simulink model "optimized_airport_sim_2"  (R2021a)
settings: Solver=VariableStepAuto  StartTime=0.0  StopTime=1e5  RelTol=1e-3
undefined symbols (not defined in the file): m, n
(part 2 of 2)

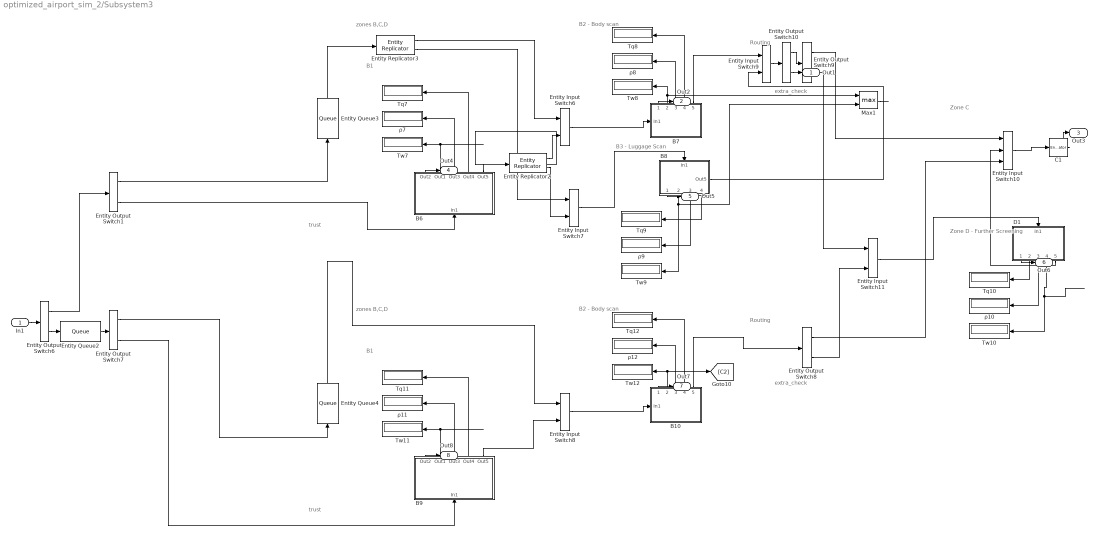
== system optimized_airport_sim_2/Subsystem3 ==
  note: B1
  note: zones B,C,D
  note: Zone C
  note: B3 -
      | Luggage
      | Scan
  note: Routing
  note: Zone D -
      |
      | Further
      | Screening
  note: B2 -
      | Body
      | scan
  note: trust
  note: extra_check
  note: B1
  note: zones B,C,D
  note: Routing
  note: B2 -
      | Body
      | scan
  note: trust
  note: extra_check
  In1 : Inport
  B10 : Subsystem
      settings: PortSchema="{\"entries\":[{\"content\":{\"sides\":[{\"content\":{\"connectorIds\":[]},\"type\":\"ConnectorPlacement.EquallySpacedRectSide\",\"uuid\":\"7ea955c4-59a0-4b16-a665-3c7419b36f79\"},{\"content\":{\"connectorIds\":[\"Out1\",\"Out2\",\"Out3\",\"Out4\",\"Out5\"],\"side\":\"RIGHT\"},\"type\":\"ConnectorPlacement.EquallySpacedRectSide\",\"uuid\":\"a8a3c229-e196-4360-bdfa-8ef645b2ce9c\"},{\"content\":{\"connectorIds\":[\"In1\"],\"side\":\"TOP\"},\"type\":\"ConnectorPlacement.EquallySpacedRectSide\",\"uuid\":\"5260f7b5-f6e8-463a-b0c5-598c56357d98\"}]},\"type\":\"ConnectorPlacement.EquallySpacedConnector\",\"uuid\":\"58c66fb9-1797-41d8-b8ed-62a065428871\"}],\"packageUris\":[\"http://schema.mathworks.com/mf0/Connector/R2020b\"],\"version\":\"1.0\"}"
  B6 : Subsystem
  B7 : Subsystem
      settings: PortSchema="{\"entries\":[{\"content\":{\"sides\":[{\"content\":{\"connectorIds\":[]},\"type\":\"ConnectorPlacement.EquallySpacedRectSide\",\"uuid\":\"7ea955c4-59a0-4b16-a665-3c7419b36f79\"},{\"content\":{\"connectorIds\":[\"Out1\",\"Out2\",\"Out3\",\"Out4\",\"Out5\"],\"side\":\"RIGHT\"},\"type\":\"ConnectorPlacement.EquallySpacedRectSide\",\"uuid\":\"a8a3c229-e196-4360-bdfa-8ef645b2ce9c\"},{\"content\":{\"connectorIds\":[\"In1\"],\"side\":\"TOP\"},\"type\":\"ConnectorPlacement.EquallySpacedRectSide\",\"uuid\":\"5260f7b5-f6e8-463a-b0c5-598c56357d98\"}]},\"type\":\"ConnectorPlacement.EquallySpacedConnector\",\"uuid\":\"58c66fb9-1797-41d8-b8ed-62a065428871\"}],\"packageUris\":[\"http://schema.mathworks.com/mf0/Connector/R2020b\"],\"version\":\"1.0\"}"
  B8 : Subsystem
      settings: PortSchema="{\"entries\":[{\"content\":{\"sides\":[{\"content\":{\"connectorIds\":[\"In1\"]},\"type\":\"ConnectorPlacement.EquallySpacedRectSide\",\"uuid\":\"7ea955c4-59a0-4b16-a665-3c7419b36f79\"},{\"content\":{\"connectorIds\":[\"Out1\",\"Out2\",\"Out3\",\"Out4\"],\"side\":\"RIGHT\"},\"type\":\"ConnectorPlacement.EquallySpacedRectSide\",\"uuid\":\"a8a3c229-e196-4360-bdfa-8ef645b2ce9c\"},{\"content\":{\"connectorIds\":[],\"side\":\"TOP\"},\"type\":\"ConnectorPlacement.EquallySpacedRectSide\",\"uuid\":\"5260f7b5-f6e8-463a-b0c5-598c56357d98\"},{\"content\":{\"connectorIds\":[\"Out5\"],\"side\":\"BOTTOM\"},\"type\":\"ConnectorPlacement.EquallySpacedRectSide\",\"uuid\":\"b778f381-c9da-4203-8e39-7c353a561693\"}]},\"type\":\"ConnectorPlacement.EquallySpacedConnector\",\"uuid\":\"58c66fb9-1797-41d8-b8ed-62a065428871\"}],\"packageUris\":[\"http://schema.mathworks.com/mf0/Connector/R2020b\"],\"version\":\"1.0\"}"
  B9 : Subsystem
  C1 : EntityTerminator  InputPortMessageModes=m  NumberEntitiesArrived=on
      settings: OutputPortMap=o0
  D1 : Subsystem
  Entity Input Switch10 : EntityInputSwitch  InputPortMessageModes=m,m,m  OutputPortMessageModes=m  NumberInputPorts=3  SwitchingCriterion=Equiprobable  Seed=450279
      settings: InputPortMap=u1,u2,u3
  Entity Input Switch11 : EntityInputSwitch  InputPortMessageModes=m,m  OutputPortMessageModes=m  SwitchingCriterion=Equiprobable  Seed=450279
  Entity Input Switch6 : EntityInputSwitch  InputPortMessageModes=m,m  OutputPortMessageModes=m
  Entity Input Switch7 : EntityInputSwitch  InputPortMessageModes=m,m  OutputPortMessageModes=m
  Entity Input Switch8 : EntityInputSwitch  InputPortMessageModes=m,m  OutputPortMessageModes=m
  Entity Input Switch9 : EntityInputSwitch  InputPortMessageModes=m,m  OutputPortMessageModes=m  ActivePortSelection=Switch  SwitchingCriterion=Equiprobable  Seed=450279
  Entity Output Switch1 : EntityOutputSwitch  InputPortMessageModes=m  OutputPortMessageModes=m,m  SwitchingCriterion=From attribute  Seed=9647085  SwitchAttributeName=trust
  Entity Output Switch10 : EntityOutputSwitch  InputPortMessageModes=m  OutputPortMessageModes=m,m  SwitchingCriterion=Equiprobable  Seed=604377
  Entity Output Switch6 : EntityOutputSwitch  InputPortMessageModes=m  OutputPortMessageModes=m,m  SwitchingCriterion=From attribute  Seed=9647085  SwitchAttributeName=luggage
  Entity Output Switch7 : EntityOutputSwitch  InputPortMessageModes=m  OutputPortMessageModes=m,m  SwitchingCriterion=From attribute  Seed=9647085  SwitchAttributeName=trust
  Entity Output Switch8 : EntityOutputSwitch  InputPortMessageModes=m  OutputPortMessageModes=m,m  SwitchingCriterion=From attribute  Seed=9632160  SwitchAttributeName=extra_check
  Entity Output Switch9 : EntityOutputSwitch  InputPortMessageModes=m  OutputPortMessageModes=m,m  SwitchingCriterion=From attribute  Seed=9632160  SwitchAttributeName=extra_check
  Entity Queue2 : Queue  InputPortMessageModes=m  OutputPortMessageModes=m  Capacity=Inf
  Entity Queue3 : Queue  InputPortMessageModes=m  OutputPortMessageModes=m  Capacity=inf
  Entity Queue4 : Queue  InputPortMessageModes=m  OutputPortMessageModes=m  Capacity=inf
  Entity Replicator2 : EntityReplicator  InputPortMessageModes=m  OutputPortMessageModes=m,m
  Entity Replicator3 : EntityReplicator  InputPortMessageModes=m  OutputPortMessageModes=m,m
  Max1 : MinMax  Function=max  Inputs=2
  Tq{7..12} (6 alike) : Display
  Tw{7..12} (6 alike) : Display
  ρ{7..12} (6 alike) : Display
  Out1 : Outport
  Out2 : Outport  Port=2
  Out3 : Outport  Port=3
  Out4 : Outport  Port=4
  Out5 : Outport  Port=5
  Out6 : Outport  Port=6
  Out7 : Outport  Port=7
  Out8 : Outport  Port=8
  wires:
  B10/4(Out4) -> Tq12/1
  B8/3(Out3) -> ρ9/1
  Entity Output Switch8/1 -> Entity Input Switch10/3
  C1/1 -> Out3/1
  Entity Output Switch1/2 -> B6/1(In1)
  Entity Input Switch10/1 -> C1/1
  B7/2(Out1) -> Tw8/1, Max1/1
  B10/5(Out5) -> Entity Output Switch8/1
  Max1/1 -> ?
  Entity Input Switch9/1 -> Entity Output Switch10/1
  Entity Output Switch9/2 -> Entity Input Switch11/1
  D1/5(Out5) -> Entity Input Switch10/2
  B8/5(Out5) -> Entity Input Switch9/2
  Entity Input Switch11/1 -> D1/1(In1)
  B9/2(Out1) -> Tw11/1
  Entity Output Switch8/2 -> Entity Input Switch11/2
  B10/3(Out3) -> ρ12/1
  B6/5(Out5) -> Entity Replicator2/1
  B10/2(Out1) -> Tw12/1, [C2]
  Entity Input Switch8/1 -> B10/1(In1)
  B9/4(Out4) -> Tq11/1
  Entity Replicator3/2 -> Entity Input Switch7/1
  D1/1(Out2) -> Out6/1
  B6/2(Out1) -> Tw7/1
  B9/3(Out3) -> ρ11/1
  B9/5(Out5) -> Entity Input Switch8/2
  Entity Queue4/1 -> Entity Input Switch8/1
  B6/1(Out2) -> Out4/1
  D1/3(Out3) -> ρ10/1
  Entity Input Switch7/1 -> B8/1(In1)
  Entity Replicator2/2 -> Entity Input Switch7/2
  D1/4(Out4) -> Tw10/1
  Entity Replicator2/1 -> Entity Input Switch6/2
  Entity Queue3/1 -> Entity Replicator3/1
  Entity Input Switch6/1 -> B7/1(In1)
  B8/1(Out2) -> Out5/1
  B8/2(Out1) -> Max1/2, Tw9/1
  Entity Replicator3/1 -> Entity Input Switch6/1
  B7/3(Out3) -> ρ8/1
  D1/2(Out1) -> Tq10/1
  B9/1(Out2) -> Out8/1
  B6/3(Out3) -> ρ7/1
  Entity Output Switch9/1 -> Entity Input Switch10/1
  B10/1(Out2) -> Out7/1
  B8/4(Out4) -> Tq9/1
  B7/5(Out5) -> Entity Input Switch9/1
  B6/4(Out4) -> Tq7/1
  Entity Output Switch10/1 -> Entity Output Switch9/1
  B7/4(Out4) -> Tq8/1
  Entity Output Switch10/2 -> Out1/1
  B7/1(Out2) -> Out2/1
  Entity Output Switch1/1 -> Entity Queue3/1
  Entity Output Switch7/1 -> Entity Queue4/1
  Entity Output Switch6/2 -> Entity Queue2/1
  Entity Output Switch6/1 -> Entity Output Switch1/1
  Entity Output Switch7/2 -> B9/1(In1)
  Entity Queue2/1 -> Entity Output Switch7/1
  In1/1 -> Entity Output Switch6/1

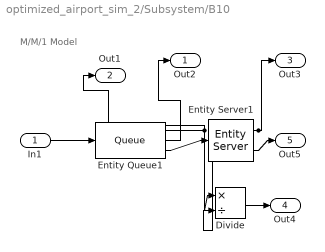
== system optimized_airport_sim_2/Subsystem/B10 ==
  note: M/M/1 Model
  In1 : Inport
  Divide : Product  Inputs=*/
  Entity Queue1 : Queue  InputPortMessageModes=m  OutputPortMessageModes=n,n,m  Capacity=inf  AverageWait=on  AverageQueueLength=on
      settings: OutputPortMap=o2,o3,o5
  Entity Server1 : EntityServer  InputPortMessageModes=m  OutputPortMessageModes=n,m  Capacity=1  ServiceTimeSource=MATLAB action  ServiceTimeAction=|  Utilization=on
      | dt = rand(1,1);
      | persistent rngInit;
      | if isempty(rngInit)
      |     seed = 7612432;
      |     rng(seed);
      |     rngInit = true;
      | end
      | 
      | % Pattern: Exponential distribution
      | mu = 7;
      | dt = -mu * log(1 - rand());
      settings: OutputPortMap=o5,o9
  Out2 : Outport
  Out1 : Outport  Port=2
  Out3 : Outport  Port=3
  Out4 : Outport  Port=4
  Out5 : Outport  Port=5
  wires:
  Divide/1 -> Out4/1
  Entity Server1/2 -> Out5/1
  Entity Queue1/3 -> Entity Server1/1
  Entity Queue1/1 -> Out1/1, Divide/1
  Entity Server1/1 -> Out3/1, Divide/2
  Entity Queue1/2 -> Out2/1
  In1/1 -> Entity Queue1/1

== system optimized_airport_sim_2/Subsystem/B6 ==
  note: M/M/1 Model
  In1 : Inport
  Divide : Product  Inputs=*/
  Entity Queue1 : Queue  InputPortMessageModes=m  OutputPortMessageModes=n,n,m  Capacity=inf  AverageWait=on  AverageQueueLength=on
      settings: OutputPortMap=o2,o3,o5
  Entity Server1 : EntityServer  InputPortMessageModes=m  OutputPortMessageModes=n,m  Capacity=1  ServiceTimeSource=MATLAB action  ServiceTimeAction=|  Utilization=on
      | dt = rand(1,1);
      | persistent rngInit;
      | if isempty(rngInit)
      |     seed = 2273520;
      |     rng(seed);
      |     rngInit = true;
      | end
      | 
      | % Pattern: Exponential distribution
      | mu = 15;
      | dt = -mu * log(1 - rand());
      settings: OutputPortMap=o5,o9
  Out2 : Outport
  Out1 : Outport  Port=2
  Out3 : Outport  Port=3
  Out4 : Outport  Port=4
  Out5 : Outport  Port=5
  wires:
  Divide/1 -> Out4/1
  Entity Server1/2 -> Out5/1
  Entity Queue1/3 -> Entity Server1/1
  Entity Queue1/1 -> Out1/1, Divide/1
  Entity Server1/1 -> Out3/1, Divide/2
  Entity Queue1/2 -> Out2/1
  In1/1 -> Entity Queue1/1

== system optimized_airport_sim_2/Subsystem/B7 ==
  note: M/M/1 Model
  In1 : Inport
  Divide : Product  Inputs=*/
  Entity Queue1 : Queue  InputPortMessageModes=m  OutputPortMessageModes=n,n,m  Capacity=inf  AverageWait=on  AverageQueueLength=on
      settings: OutputPortMap=o2,o3,o5
  Entity Server1 : EntityServer  InputPortMessageModes=m  OutputPortMessageModes=n,m  Capacity=1  ServiceTimeSource=MATLAB action  ServiceTimeAction=|  Utilization=on
      | dt = rand(1,1);
      | persistent rngInit;
      | if isempty(rngInit)
      |     seed = 7612432;
      |     rng(seed);
      |     rngInit = true;
      | end
      | 
      | % Pattern: Exponential distribution
      | mu = 7;
      | dt = -mu * log(1 - rand());
      settings: OutputPortMap=o5,o9
  Out2 : Outport
  Out1 : Outport  Port=2
  Out3 : Outport  Port=3
  Out4 : Outport  Port=4
  Out5 : Outport  Port=5
  wires:
  In1/1 -> Entity Queue1/1
  Entity Queue1/2 -> Out2/1
  Entity Server1/1 -> Divide/2, Out3/1
  Entity Queue1/1 -> Divide/1, Out1/1
  Entity Queue1/3 -> Entity Server1/1
  Entity Server1/2 -> Out5/1
  Divide/1 -> Out4/1

== system optimized_airport_sim_2/Subsystem/B8 ==
  note: M/M/1 Model
  In1 : Inport
  Divide : Product  Inputs=*/
  Entity Queue1 : Queue  InputPortMessageModes=m  OutputPortMessageModes=n,n,m  Capacity=inf  AverageWait=on  AverageQueueLength=on
      settings: OutputPortMap=o2,o3,o5
  Entity Server1 : EntityServer  InputPortMessageModes=m  OutputPortMessageModes=n,m  Capacity=1  ServiceTimeSource=MATLAB action  ServiceTimeAction=|  Utilization=on
      | dt = rand(1,1);
      | persistent rngInit;
      | if isempty(rngInit)
      |     seed = 6069205;
      |     rng(seed);
      |     rngInit = true;
      | end
      | 
      | % Pattern: Exponential distribution
      | mu = 8;
      | dt = -mu * log(1 - rand());
      settings: OutputPortMap=o5,o9
  Out2 : Outport
  Out1 : Outport  Port=2
  Out3 : Outport  Port=3
  Out4 : Outport  Port=4
  Out5 : Outport  Port=5
  wires:
  Divide/1 -> Out4/1
  Entity Server1/2 -> Out5/1
  Entity Queue1/3 -> Entity Server1/1
  Entity Queue1/1 -> Out1/1, Divide/1
  Entity Server1/1 -> Out3/1, Divide/2
  Entity Queue1/2 -> Out2/1
  In1/1 -> Entity Queue1/1

== system optimized_airport_sim_2/Subsystem/B9 ==
  note: M/M/1 Model
  In1 : Inport
  Divide : Product  Inputs=*/
  Entity Queue1 : Queue  InputPortMessageModes=m  OutputPortMessageModes=n,n,m  Capacity=inf  AverageWait=on  AverageQueueLength=on
      settings: OutputPortMap=o2,o3,o5
  Entity Server1 : EntityServer  InputPortMessageModes=m  OutputPortMessageModes=n,m  Capacity=1  ServiceTimeSource=MATLAB action  ServiceTimeAction=|  Utilization=on
      | dt = rand(1,1);
      | persistent rngInit;
      | if isempty(rngInit)
      |     seed = 2273520;
      |     rng(seed);
      |     rngInit = true;
      | end
      | 
      | % Pattern: Exponential distribution
      | mu = 10;
      | dt = -mu * log(1 - rand());
      settings: OutputPortMap=o5,o9
  Out2 : Outport
  Out1 : Outport  Port=2
  Out3 : Outport  Port=3
  Out4 : Outport  Port=4
  Out5 : Outport  Port=5
  wires:
  In1/1 -> Entity Queue1/1
  Entity Queue1/2 -> Out2/1
  Entity Server1/1 -> Divide/2, Out3/1
  Entity Queue1/1 -> Divide/1, Out1/1
  Entity Queue1/3 -> Entity Server1/1
  Entity Server1/2 -> Out5/1
  Divide/1 -> Out4/1

== system optimized_airport_sim_2/Subsystem/D1 ==
  note: M/M/1 Model
  In1 : Inport
  Divide : Product  Inputs=*/
  Entity Queue1 : Queue  InputPortMessageModes=m  OutputPortMessageModes=n,n,m  Capacity=inf  AverageWait=on  AverageQueueLength=on
      settings: OutputPortMap=o2,o3,o5
  Entity Server1 : EntityServer  InputPortMessageModes=m  OutputPortMessageModes=n,m  Capacity=1  ServiceTimeSource=MATLAB action  ServiceTimeAction=|  Utilization=on
      | dt = rand(1,1);
      | persistent rngInit;
      | if isempty(rngInit)
      |     seed = 6069205;
      |     rng(seed);
      |     rngInit = true;
      | end
      | 
      | % Pattern: Exponential distribution
      | mu = 60*3;
      | dt = -mu * log(1 - rand());
      settings: OutputPortMap=o5,o9
  Out2 : Outport
  Out1 : Outport  Port=2
  Out3 : Outport  Port=3
  Out4 : Outport  Port=4
  Out5 : Outport  Port=5
  wires:
  In1/1 -> Entity Queue1/1
  Entity Queue1/2 -> Out2/1
  Entity Server1/1 -> Divide/2, Out3/1
  Entity Queue1/1 -> Divide/1, Out1/1
  Entity Queue1/3 -> Entity Server1/1
  Entity Server1/2 -> Out5/1
  Divide/1 -> Out4/1

== system optimized_airport_sim_2/Subsystem1/B10 ==
  note: M/M/1 Model
  In1 : Inport
  Divide : Product  Inputs=*/
  Entity Queue1 : Queue  InputPortMessageModes=m  OutputPortMessageModes=n,n,m  Capacity=inf  AverageWait=on  AverageQueueLength=on
      settings: OutputPortMap=o2,o3,o5
  Entity Server1 : EntityServer  InputPortMessageModes=m  OutputPortMessageModes=n,m  Capacity=1  ServiceTimeSource=MATLAB action  ServiceTimeAction=|  Utilization=on
      | dt = rand(1,1);
      | persistent rngInit;
      | if isempty(rngInit)
      |     seed = 7612432;
      |     rng(seed);
      |     rngInit = true;
      | end
      | 
      | % Pattern: Exponential distribution
      | mu = 7;
      | dt = -mu * log(1 - rand());
      settings: OutputPortMap=o5,o9
  Out2 : Outport
  Out1 : Outport  Port=2
  Out3 : Outport  Port=3
  Out4 : Outport  Port=4
  Out5 : Outport  Port=5
  wires:
  In1/1 -> Entity Queue1/1
  Entity Queue1/2 -> Out2/1
  Entity Server1/1 -> Divide/2, Out3/1
  Entity Queue1/1 -> Divide/1, Out1/1
  Entity Queue1/3 -> Entity Server1/1
  Entity Server1/2 -> Out5/1
  Divide/1 -> Out4/1

== system optimized_airport_sim_2/Subsystem1/B6 ==
  note: M/M/1 Model
  In1 : Inport
  Divide : Product  Inputs=*/
  Entity Queue1 : Queue  InputPortMessageModes=m  OutputPortMessageModes=n,n,m  Capacity=inf  AverageWait=on  AverageQueueLength=on
      settings: OutputPortMap=o2,o3,o5
  Entity Server1 : EntityServer  InputPortMessageModes=m  OutputPortMessageModes=n,m  Capacity=1  ServiceTimeSource=MATLAB action  ServiceTimeAction=|  Utilization=on
      | dt = rand(1,1);
      | persistent rngInit;
      | if isempty(rngInit)
      |     seed = 2273520;
      |     rng(seed);
      |     rngInit = true;
      | end
      | 
      | % Pattern: Exponential distribution
      | mu = 15;
      | dt = -mu * log(1 - rand());
      settings: OutputPortMap=o5,o9
  Out2 : Outport
  Out1 : Outport  Port=2
  Out3 : Outport  Port=3
  Out4 : Outport  Port=4
  Out5 : Outport  Port=5
  wires:
  In1/1 -> Entity Queue1/1
  Entity Queue1/2 -> Out2/1
  Entity Server1/1 -> Divide/2, Out3/1
  Entity Queue1/1 -> Divide/1, Out1/1
  Entity Queue1/3 -> Entity Server1/1
  Entity Server1/2 -> Out5/1
  Divide/1 -> Out4/1

== system optimized_airport_sim_2/Subsystem1/B7 ==
  note: M/M/1 Model
  In1 : Inport
  Divide : Product  Inputs=*/
  Entity Queue1 : Queue  InputPortMessageModes=m  OutputPortMessageModes=n,n,m  Capacity=inf  AverageWait=on  AverageQueueLength=on
      settings: OutputPortMap=o2,o3,o5
  Entity Server1 : EntityServer  InputPortMessageModes=m  OutputPortMessageModes=n,m  Capacity=1  ServiceTimeSource=MATLAB action  ServiceTimeAction=|  Utilization=on
      | dt = rand(1,1);
      | persistent rngInit;
      | if isempty(rngInit)
      |     seed = 7612432;
      |     rng(seed);
      |     rngInit = true;
      | end
      | 
      | % Pattern: Exponential distribution
      | mu = 7;
      | dt = -mu * log(1 - rand());
      settings: OutputPortMap=o5,o9
  Out2 : Outport
  Out1 : Outport  Port=2
  Out3 : Outport  Port=3
  Out4 : Outport  Port=4
  Out5 : Outport  Port=5
  wires:
  Divide/1 -> Out4/1
  Entity Server1/2 -> Out5/1
  Entity Queue1/3 -> Entity Server1/1
  Entity Queue1/1 -> Out1/1, Divide/1
  Entity Server1/1 -> Out3/1, Divide/2
  Entity Queue1/2 -> Out2/1
  In1/1 -> Entity Queue1/1

== system optimized_airport_sim_2/Subsystem1/B8 ==
  note: M/M/1 Model
  In1 : Inport
  Divide : Product  Inputs=*/
  Entity Queue1 : Queue  InputPortMessageModes=m  OutputPortMessageModes=n,n,m  Capacity=inf  AverageWait=on  AverageQueueLength=on
      settings: OutputPortMap=o2,o3,o5
  Entity Server1 : EntityServer  InputPortMessageModes=m  OutputPortMessageModes=n,m  Capacity=1  ServiceTimeSource=MATLAB action  ServiceTimeAction=|  Utilization=on
      | dt = rand(1,1);
      | persistent rngInit;
      | if isempty(rngInit)
      |     seed = 6069205;
      |     rng(seed);
      |     rngInit = true;
      | end
      | 
      | % Pattern: Exponential distribution
      | mu = 8;
      | dt = -mu * log(1 - rand());
      settings: OutputPortMap=o5,o9
  Out2 : Outport
  Out1 : Outport  Port=2
  Out3 : Outport  Port=3
  Out4 : Outport  Port=4
  Out5 : Outport  Port=5
  wires:
  In1/1 -> Entity Queue1/1
  Entity Queue1/2 -> Out2/1
  Entity Server1/1 -> Divide/2, Out3/1
  Entity Queue1/1 -> Divide/1, Out1/1
  Entity Queue1/3 -> Entity Server1/1
  Entity Server1/2 -> Out5/1
  Divide/1 -> Out4/1

== system optimized_airport_sim_2/Subsystem1/B9 ==
  note: M/M/1 Model
  In1 : Inport
  Divide : Product  Inputs=*/
  Entity Queue1 : Queue  InputPortMessageModes=m  OutputPortMessageModes=n,n,m  Capacity=inf  AverageWait=on  AverageQueueLength=on
      settings: OutputPortMap=o2,o3,o5
  Entity Server1 : EntityServer  InputPortMessageModes=m  OutputPortMessageModes=n,m  Capacity=1  ServiceTimeSource=MATLAB action  ServiceTimeAction=|  Utilization=on
      | dt = rand(1,1);
      | persistent rngInit;
      | if isempty(rngInit)
      |     seed = 2273520;
      |     rng(seed);
      |     rngInit = true;
      | end
      | 
      | % Pattern: Exponential distribution
      | mu = 10;
      | dt = -mu * log(1 - rand());
      settings: OutputPortMap=o5,o9
  Out2 : Outport
  Out1 : Outport  Port=2
  Out3 : Outport  Port=3
  Out4 : Outport  Port=4
  Out5 : Outport  Port=5
  wires:
  Divide/1 -> Out4/1
  Entity Server1/2 -> Out5/1
  Entity Queue1/3 -> Entity Server1/1
  Entity Queue1/1 -> Out1/1, Divide/1
  Entity Server1/1 -> Out3/1, Divide/2
  Entity Queue1/2 -> Out2/1
  In1/1 -> Entity Queue1/1

== system optimized_airport_sim_2/Subsystem1/D1 ==
  note: M/M/1 Model
  In1 : Inport
  Divide : Product  Inputs=*/
  Entity Queue1 : Queue  InputPortMessageModes=m  OutputPortMessageModes=n,n,m  Capacity=inf  AverageWait=on  AverageQueueLength=on
      settings: OutputPortMap=o2,o3,o5
  Entity Server1 : EntityServer  InputPortMessageModes=m  OutputPortMessageModes=n,m  Capacity=1  ServiceTimeSource=MATLAB action  ServiceTimeAction=|  Utilization=on
      | dt = rand(1,1);
      | persistent rngInit;
      | if isempty(rngInit)
      |     seed = 6069205;
      |     rng(seed);
      |     rngInit = true;
      | end
      | 
      | % Pattern: Exponential distribution
      | mu = 60*3;
      | dt = -mu * log(1 - rand());
      settings: OutputPortMap=o5,o9
  Out2 : Outport
  Out1 : Outport  Port=2
  Out3 : Outport  Port=3
  Out4 : Outport  Port=4
  Out5 : Outport  Port=5
  wires:
  Divide/1 -> Out4/1
  Entity Server1/2 -> Out5/1
  Entity Queue1/3 -> Entity Server1/1
  Entity Queue1/1 -> Out1/1, Divide/1
  Entity Server1/1 -> Out3/1, Divide/2
  Entity Queue1/2 -> Out2/1
  In1/1 -> Entity Queue1/1

== system optimized_airport_sim_2/Subsystem2/B10 ==
  note: M/M/1 Model
  In1 : Inport
  Divide : Product  Inputs=*/
  Entity Queue1 : Queue  InputPortMessageModes=m  OutputPortMessageModes=n,n,m  Capacity=inf  AverageWait=on  AverageQueueLength=on
      settings: OutputPortMap=o2,o3,o5
  Entity Server1 : EntityServer  InputPortMessageModes=m  OutputPortMessageModes=n,m  Capacity=1  ServiceTimeSource=MATLAB action  ServiceTimeAction=|  Utilization=on
      | dt = rand(1,1);
      | persistent rngInit;
      | if isempty(rngInit)
      |     seed = 7612432;
      |     rng(seed);
      |     rngInit = true;
      | end
      | 
      | % Pattern: Exponential distribution
      | mu = 7;
      | dt = -mu * log(1 - rand());
      settings: OutputPortMap=o5,o9
  Out2 : Outport
  Out1 : Outport  Port=2
  Out3 : Outport  Port=3
  Out4 : Outport  Port=4
  Out5 : Outport  Port=5
  wires:
  In1/1 -> Entity Queue1/1
  Entity Queue1/2 -> Out2/1
  Entity Server1/1 -> Divide/2, Out3/1
  Entity Queue1/1 -> Divide/1, Out1/1
  Entity Queue1/3 -> Entity Server1/1
  Entity Server1/2 -> Out5/1
  Divide/1 -> Out4/1

== system optimized_airport_sim_2/Subsystem2/B6 ==
  note: M/M/1 Model
  In1 : Inport
  Divide : Product  Inputs=*/
  Entity Queue1 : Queue  InputPortMessageModes=m  OutputPortMessageModes=n,n,m  Capacity=inf  AverageWait=on  AverageQueueLength=on
      settings: OutputPortMap=o2,o3,o5
  Entity Server1 : EntityServer  InputPortMessageModes=m  OutputPortMessageModes=n,m  Capacity=1  ServiceTimeSource=MATLAB action  ServiceTimeAction=|  Utilization=on
      | dt = rand(1,1);
      | persistent rngInit;
      | if isempty(rngInit)
      |     seed = 2273520;
      |     rng(seed);
      |     rngInit = true;
      | end
      | 
      | % Pattern: Exponential distribution
      | mu = 15;
      | dt = -mu * log(1 - rand());
      settings: OutputPortMap=o5,o9
  Out2 : Outport
  Out1 : Outport  Port=2
  Out3 : Outport  Port=3
  Out4 : Outport  Port=4
  Out5 : Outport  Port=5
  wires:
  In1/1 -> Entity Queue1/1
  Entity Queue1/2 -> Out2/1
  Entity Server1/1 -> Divide/2, Out3/1
  Entity Queue1/1 -> Divide/1, Out1/1
  Entity Queue1/3 -> Entity Server1/1
  Entity Server1/2 -> Out5/1
  Divide/1 -> Out4/1

== system optimized_airport_sim_2/Subsystem2/B7 ==
  note: M/M/1 Model
  In1 : Inport
  Divide : Product  Inputs=*/
  Entity Queue1 : Queue  InputPortMessageModes=m  OutputPortMessageModes=n,n,m  Capacity=inf  AverageWait=on  AverageQueueLength=on
      settings: OutputPortMap=o2,o3,o5
  Entity Server1 : EntityServer  InputPortMessageModes=m  OutputPortMessageModes=n,m  Capacity=1  ServiceTimeSource=MATLAB action  ServiceTimeAction=|  Utilization=on
      | dt = rand(1,1);
      | persistent rngInit;
      | if isempty(rngInit)
      |     seed = 7612432;
      |     rng(seed);
      |     rngInit = true;
      | end
      | 
      | % Pattern: Exponential distribution
      | mu = 7;
      | dt = -mu * log(1 - rand());
      settings: OutputPortMap=o5,o9
  Out2 : Outport
  Out1 : Outport  Port=2
  Out3 : Outport  Port=3
  Out4 : Outport  Port=4
  Out5 : Outport  Port=5
  wires:
  Divide/1 -> Out4/1
  Entity Server1/2 -> Out5/1
  Entity Queue1/3 -> Entity Server1/1
  Entity Queue1/1 -> Out1/1, Divide/1
  Entity Server1/1 -> Out3/1, Divide/2
  Entity Queue1/2 -> Out2/1
  In1/1 -> Entity Queue1/1

== system optimized_airport_sim_2/Subsystem2/B8 ==
  note: M/M/1 Model
  In1 : Inport
  Divide : Product  Inputs=*/
  Entity Queue1 : Queue  InputPortMessageModes=m  OutputPortMessageModes=n,n,m  Capacity=inf  AverageWait=on  AverageQueueLength=on
      settings: OutputPortMap=o2,o3,o5
  Entity Server1 : EntityServer  InputPortMessageModes=m  OutputPortMessageModes=n,m  Capacity=1  ServiceTimeSource=MATLAB action  ServiceTimeAction=|  Utilization=on
      | dt = rand(1,1);
      | persistent rngInit;
      | if isempty(rngInit)
      |     seed = 6069205;
      |     rng(seed);
      |     rngInit = true;
      | end
      | 
      | % Pattern: Exponential distribution
      | mu = 8;
      | dt = -mu * log(1 - rand());
      settings: OutputPortMap=o5,o9
  Out2 : Outport
  Out1 : Outport  Port=2
  Out3 : Outport  Port=3
  Out4 : Outport  Port=4
  Out5 : Outport  Port=5
  wires:
  In1/1 -> Entity Queue1/1
  Entity Queue1/2 -> Out2/1
  Entity Server1/1 -> Divide/2, Out3/1
  Entity Queue1/1 -> Divide/1, Out1/1
  Entity Queue1/3 -> Entity Server1/1
  Entity Server1/2 -> Out5/1
  Divide/1 -> Out4/1

== system optimized_airport_sim_2/Subsystem2/B9 ==
  note: M/M/1 Model
  In1 : Inport
  Divide : Product  Inputs=*/
  Entity Queue1 : Queue  InputPortMessageModes=m  OutputPortMessageModes=n,n,m  Capacity=inf  AverageWait=on  AverageQueueLength=on
      settings: OutputPortMap=o2,o3,o5
  Entity Server1 : EntityServer  InputPortMessageModes=m  OutputPortMessageModes=n,m  Capacity=1  ServiceTimeSource=MATLAB action  ServiceTimeAction=|  Utilization=on
      | dt = rand(1,1);
      | persistent rngInit;
      | if isempty(rngInit)
      |     seed = 2273520;
      |     rng(seed);
      |     rngInit = true;
      | end
      | 
      | % Pattern: Exponential distribution
      | mu = 10;
      | dt = -mu * log(1 - rand());
      settings: OutputPortMap=o5,o9
  Out2 : Outport
  Out1 : Outport  Port=2
  Out3 : Outport  Port=3
  Out4 : Outport  Port=4
  Out5 : Outport  Port=5
  wires:
  Divide/1 -> Out4/1
  Entity Server1/2 -> Out5/1
  Entity Queue1/3 -> Entity Server1/1
  Entity Queue1/1 -> Out1/1, Divide/1
  Entity Server1/1 -> Out3/1, Divide/2
  Entity Queue1/2 -> Out2/1
  In1/1 -> Entity Queue1/1

== system optimized_airport_sim_2/Subsystem2/D1 ==
  note: M/M/1 Model
  In1 : Inport
  Divide : Product  Inputs=*/
  Entity Queue1 : Queue  InputPortMessageModes=m  OutputPortMessageModes=n,n,m  Capacity=inf  AverageWait=on  AverageQueueLength=on
      settings: OutputPortMap=o2,o3,o5
  Entity Server1 : EntityServer  InputPortMessageModes=m  OutputPortMessageModes=n,m  Capacity=1  ServiceTimeSource=MATLAB action  ServiceTimeAction=|  Utilization=on
      | dt = rand(1,1);
      | persistent rngInit;
      | if isempty(rngInit)
      |     seed = 6069205;
      |     rng(seed);
      |     rngInit = true;
      | end
      | 
      | % Pattern: Exponential distribution
      | mu = 60*3;
      | dt = -mu * log(1 - rand());
      settings: OutputPortMap=o5,o9
  Out2 : Outport
  Out1 : Outport  Port=2
  Out3 : Outport  Port=3
  Out4 : Outport  Port=4
  Out5 : Outport  Port=5
  wires:
  Divide/1 -> Out4/1
  Entity Server1/2 -> Out5/1
  Entity Queue1/3 -> Entity Server1/1
  Entity Queue1/1 -> Out1/1, Divide/1
  Entity Server1/1 -> Out3/1, Divide/2
  Entity Queue1/2 -> Out2/1
  In1/1 -> Entity Queue1/1

== system optimized_airport_sim_2/Subsystem3/B10 ==
  note: M/M/1 Model
  In1 : Inport
  Divide : Product  Inputs=*/
  Entity Queue1 : Queue  InputPortMessageModes=m  OutputPortMessageModes=n,n,m  Capacity=inf  AverageWait=on  AverageQueueLength=on
      settings: OutputPortMap=o2,o3,o5
  Entity Server1 : EntityServer  InputPortMessageModes=m  OutputPortMessageModes=n,m  Capacity=1  ServiceTimeSource=MATLAB action  ServiceTimeAction=|  Utilization=on
      | dt = rand(1,1);
      | persistent rngInit;
      | if isempty(rngInit)
      |     seed = 7612432;
      |     rng(seed);
      |     rngInit = true;
      | end
      | 
      | % Pattern: Exponential distribution
      | mu = 7;
      | dt = -mu * log(1 - rand());
      settings: OutputPortMap=o5,o9
  Out2 : Outport
  Out1 : Outport  Port=2
  Out3 : Outport  Port=3
  Out4 : Outport  Port=4
  Out5 : Outport  Port=5
  wires:
  Divide/1 -> Out4/1
  Entity Server1/2 -> Out5/1
  Entity Queue1/3 -> Entity Server1/1
  Entity Queue1/1 -> Out1/1, Divide/1
  Entity Server1/1 -> Out3/1, Divide/2
  Entity Queue1/2 -> Out2/1
  In1/1 -> Entity Queue1/1

== system optimized_airport_sim_2/Subsystem3/B6 ==
  note: M/M/1 Model
  In1 : Inport
  Divide : Product  Inputs=*/
  Entity Queue1 : Queue  InputPortMessageModes=m  OutputPortMessageModes=n,n,m  Capacity=inf  AverageWait=on  AverageQueueLength=on
      settings: OutputPortMap=o2,o3,o5
  Entity Server1 : EntityServer  InputPortMessageModes=m  OutputPortMessageModes=n,m  Capacity=1  ServiceTimeSource=MATLAB action  ServiceTimeAction=|  Utilization=on
      | dt = rand(1,1);
      | persistent rngInit;
      | if isempty(rngInit)
      |     seed = 2273520;
      |     rng(seed);
      |     rngInit = true;
      | end
      | 
      | % Pattern: Exponential distribution
      | mu = 15;
      | dt = -mu * log(1 - rand());
      settings: OutputPortMap=o5,o9
  Out2 : Outport
  Out1 : Outport  Port=2
  Out3 : Outport  Port=3
  Out4 : Outport  Port=4
  Out5 : Outport  Port=5
  wires:
  Divide/1 -> Out4/1
  Entity Server1/2 -> Out5/1
  Entity Queue1/3 -> Entity Server1/1
  Entity Queue1/1 -> Out1/1, Divide/1
  Entity Server1/1 -> Out3/1, Divide/2
  Entity Queue1/2 -> Out2/1
  In1/1 -> Entity Queue1/1

== system optimized_airport_sim_2/Subsystem3/B7 ==
  note: M/M/1 Model
  In1 : Inport
  Divide : Product  Inputs=*/
  Entity Queue1 : Queue  InputPortMessageModes=m  OutputPortMessageModes=n,n,m  Capacity=inf  AverageWait=on  AverageQueueLength=on
      settings: OutputPortMap=o2,o3,o5
  Entity Server1 : EntityServer  InputPortMessageModes=m  OutputPortMessageModes=n,m  Capacity=1  ServiceTimeSource=MATLAB action  ServiceTimeAction=|  Utilization=on
      | dt = rand(1,1);
      | persistent rngInit;
      | if isempty(rngInit)
      |     seed = 7612432;
      |     rng(seed);
      |     rngInit = true;
      | end
      | 
      | % Pattern: Exponential distribution
      | mu = 7;
      | dt = -mu * log(1 - rand());
      settings: OutputPortMap=o5,o9
  Out2 : Outport
  Out1 : Outport  Port=2
  Out3 : Outport  Port=3
  Out4 : Outport  Port=4
  Out5 : Outport  Port=5
  wires:
  In1/1 -> Entity Queue1/1
  Entity Queue1/2 -> Out2/1
  Entity Server1/1 -> Divide/2, Out3/1
  Entity Queue1/1 -> Divide/1, Out1/1
  Entity Queue1/3 -> Entity Server1/1
  Entity Server1/2 -> Out5/1
  Divide/1 -> Out4/1

== system optimized_airport_sim_2/Subsystem3/B8 ==
  note: M/M/1 Model
  In1 : Inport
  Divide : Product  Inputs=*/
  Entity Queue1 : Queue  InputPortMessageModes=m  OutputPortMessageModes=n,n,m  Capacity=inf  AverageWait=on  AverageQueueLength=on
      settings: OutputPortMap=o2,o3,o5
  Entity Server1 : EntityServer  InputPortMessageModes=m  OutputPortMessageModes=n,m  Capacity=1  ServiceTimeSource=MATLAB action  ServiceTimeAction=|  Utilization=on
      | dt = rand(1,1);
      | persistent rngInit;
      | if isempty(rngInit)
      |     seed = 6069205;
      |     rng(seed);
      |     rngInit = true;
      | end
      | 
      | % Pattern: Exponential distribution
      | mu = 8;
      | dt = -mu * log(1 - rand());
      settings: OutputPortMap=o5,o9
  Out2 : Outport
  Out1 : Outport  Port=2
  Out3 : Outport  Port=3
  Out4 : Outport  Port=4
  Out5 : Outport  Port=5
  wires:
  Divide/1 -> Out4/1
  Entity Server1/2 -> Out5/1
  Entity Queue1/3 -> Entity Server1/1
  Entity Queue1/1 -> Out1/1, Divide/1
  Entity Server1/1 -> Out3/1, Divide/2
  Entity Queue1/2 -> Out2/1
  In1/1 -> Entity Queue1/1

== system optimized_airport_sim_2/Subsystem3/B9 ==
  note: M/M/1 Model
  In1 : Inport
  Divide : Product  Inputs=*/
  Entity Queue1 : Queue  InputPortMessageModes=m  OutputPortMessageModes=n,n,m  Capacity=inf  AverageWait=on  AverageQueueLength=on
      settings: OutputPortMap=o2,o3,o5
  Entity Server1 : EntityServer  InputPortMessageModes=m  OutputPortMessageModes=n,m  Capacity=1  ServiceTimeSource=MATLAB action  ServiceTimeAction=|  Utilization=on
      | dt = rand(1,1);
      | persistent rngInit;
      | if isempty(rngInit)
      |     seed = 2273520;
      |     rng(seed);
      |     rngInit = true;
      | end
      | 
      | % Pattern: Exponential distribution
      | mu = 10;
      | dt = -mu * log(1 - rand());
      settings: OutputPortMap=o5,o9
  Out2 : Outport
  Out1 : Outport  Port=2
  Out3 : Outport  Port=3
  Out4 : Outport  Port=4
  Out5 : Outport  Port=5
  wires:
  In1/1 -> Entity Queue1/1
  Entity Queue1/2 -> Out2/1
  Entity Server1/1 -> Divide/2, Out3/1
  Entity Queue1/1 -> Divide/1, Out1/1
  Entity Queue1/3 -> Entity Server1/1
  Entity Server1/2 -> Out5/1
  Divide/1 -> Out4/1

== system optimized_airport_sim_2/Subsystem3/D1 ==
  note: M/M/1 Model
  In1 : Inport
  Divide : Product  Inputs=*/
  Entity Queue1 : Queue  InputPortMessageModes=m  OutputPortMessageModes=n,n,m  Capacity=inf  AverageWait=on  AverageQueueLength=on
      settings: OutputPortMap=o2,o3,o5
  Entity Server1 : EntityServer  InputPortMessageModes=m  OutputPortMessageModes=n,m  Capacity=1  ServiceTimeSource=MATLAB action  ServiceTimeAction=|  Utilization=on
      | dt = rand(1,1);
      | persistent rngInit;
      | if isempty(rngInit)
      |     seed = 6069205;
      |     rng(seed);
      |     rngInit = true;
      | end
      | 
      | % Pattern: Exponential distribution
      | mu = 60*3;
      | dt = -mu * log(1 - rand());
      settings: OutputPortMap=o5,o9
  Out2 : Outport
  Out1 : Outport  Port=2
  Out3 : Outport  Port=3
  Out4 : Outport  Port=4
  Out5 : Outport  Port=5
  wires:
  In1/1 -> Entity Queue1/1
  Entity Queue1/2 -> Out2/1
  Entity Server1/1 -> Divide/2, Out3/1
  Entity Queue1/1 -> Divide/1, Out1/1
  Entity Queue1/3 -> Entity Server1/1
  Entity Server1/2 -> Out5/1
  Divide/1 -> Out4/1
